simulink model "current_measure"  (Simulink 8.1)
settings: Solver=ode45  StartTime=0.0  StopTime=10.0  RelTol=1e-3
settings Model: Creator=hlopez5  LastModifiedBy=hlopez5
settings DataIOCC: SignalLoggingSaveFormat=Dataset
settings OptimizationCC: ExpressionDepthLimit=128
settings DebuggingCC: FcnCallInpInsideContextMsg=EnableAllAsError
settings GRTTargetCC: CombineOutputUpdateFcns=on  GRTInterface=off

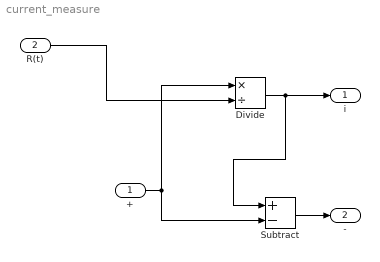
== system current_measure ==
  + : Inport
  R(t) : Inport  Port=2
  Divide : Product  Inputs=*/
  Subtract : Sum  Inputs=+-
  i : Outport
  - : Outport  Port=2
  wires:
  +/1 -> Subtract/2, Divide/1
  R(t)/1 -> Divide/2
  Divide/1 -> Subtract/1, i/1
  Subtract/1 -> -/1
